simulink library "led_control"  (R2023b)
settings: Solver=VariableStepAuto  StartTime=0.0  StopTime=10.0  RelTol=1e-3
libraries: $bdroot x1
settings Model: Creator=Professional  LastModifiedBy=Olga
settings SFSimCC: SimCustomHeaderCode="#include \"led_control.h\""  SimUserSources=.\led_control.c  SimAnalyzeCustomCode=on
settings RTWCC: RTWUseSimCustomCode=on  CustomHeaderCode="#include \"led_control.h\""  CustomSource=.\led_control.c

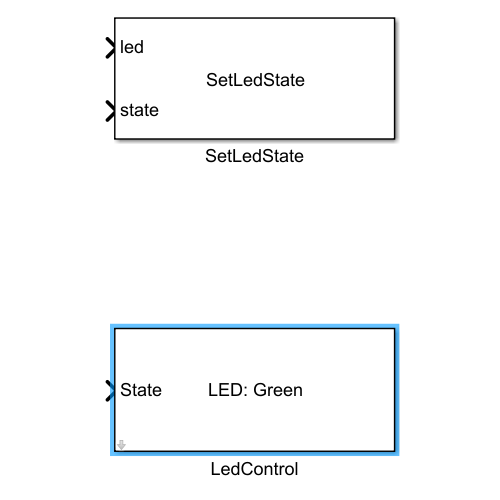
[thumbnail: Simulink's stored preview of the top-level diagram]
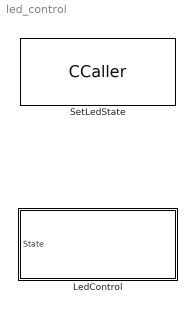
== system led_control ==
  LedControl : Subsystem  mask{Led=Green}
      mask init:
      | maskObj = Simulink.Mask.get(gcb);
      | ledName = maskObj.getParameter('Led').Value;
      | 
      | blockName = "LED: " + ledName;
      mask TypeOptions Led: Green | Blue | Red
      mask Display:
      | disp(blockName);
      | port_label('input', 1, 'State');
  SetLedState : CCaller  FunctionName=SetLedState  PortSpecificationStruct="%)30     .    R ,   8    (     @         %    \"     (    !     0         %  0 \"0    $    _    07)G3F%M90  4&]R=$YA;64 4V-O<&4     26YD97@     5'EP90      4VEZ90      27-';&]B86P   X    P    !@    @    $          4    (     0    ,    !         !   P!L960 #@   #     &    \"     0         !0    @    !     P    $         $  # &QE9  .    .     8    (    !          %    \"     $    %     0         0    !0   $EN<'5T    #@   #@    &    \"     8         !0    @    !     0    $         \"0    @               X    X    !@    @    $          4    (     0    4    !         !     %    =6EN=#@    .    ,     8    (    !          %    \"     $    !     0         0  $ ,0    X    P    !@    @    ) @        4    (     0    $    !          (  0      #@   #@    &    \"     0         !0    @    !    !0    $         $     4   !S=&%T90    X    X    !@    @    $          4    (     0    4    !         !     %    <W1A=&4    .    .     8    (    !          %    \"     $    %     0         0    !0   $EN<'5T    #@   #@    &    \"     8         !0    @    !     0    $         \"0    @           #P/PX    X    !@    @    $          4    (     0    4    !         !     %    =6EN=#@    .    ,     8    (    !          %    \"     $    !     0         0  $ ,0    X    P    !@    @    ) @        4    (     0    $    !          (  0"

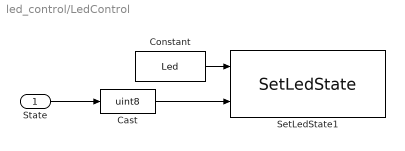
== system led_control/LedControl ==
  State : Inport  OutDataTypeStr=boolean
  Cast : DataTypeConversion  OutDataTypeStr=uint8  RndMeth=Simplest  SaturateOnIntegerOverflow=off
  Constant : Constant  Value=Led  OutDataTypeStr=uint8
  SetLedState1 : $bdroot/SetLedState  SampleTime=-1
  wires:
  Constant/1 -> SetLedState1/1
  State/1 -> Cast/1
  Cast/1 -> SetLedState1/2
